simulink model "robotCICESEneurSECcorrGamGA3Wvlt2"  (R2015a)
settings: Solver=ode5  StartTime=0.0  StopTime=200  FixedStep=2.5e-4  MinStep=2.5e-5  RelTol=1e-3
undefined symbols (not defined in the file): F1, F10, F11, F12, F13, F14, F15, F16, F17, F18, F19, F2, F20, F3, F4, F5, F6, F7, F8, F9, Vfinal, Wfinal
libraries: fuzblock x2, simulink_extras x2, simulink x1
settings Model: SimulationMode=accelerator  CovSFcnEnable=off  Creator=Andres Othon  LastModifiedBy=Elothron02
settings DataIOCC: LimitDataPoints=off
settings DebuggingCC: SolverPrmCheckMsg=warning

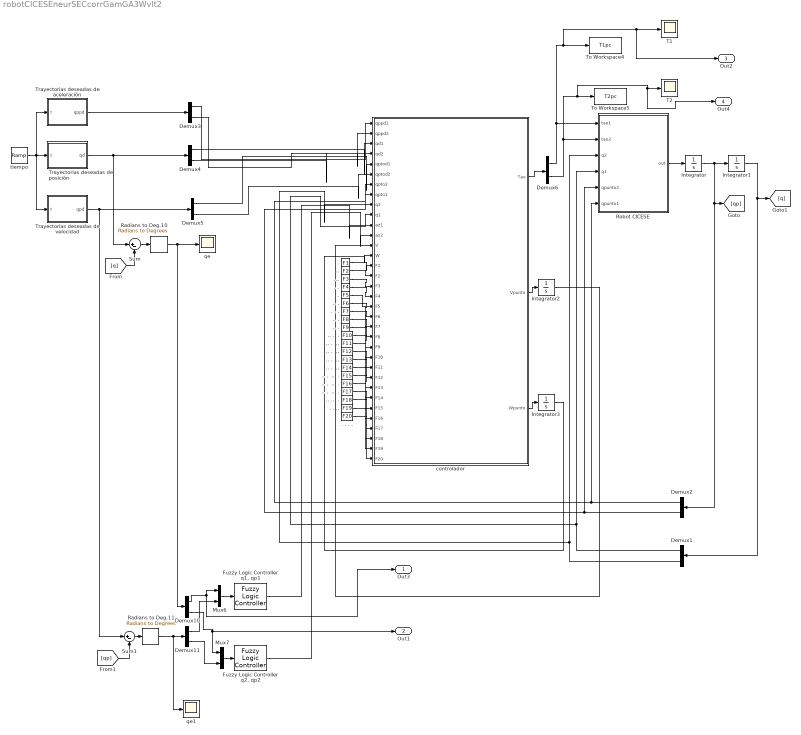
== system robotCICESEneurSECcorrGamGA3Wvlt2 ==
  . : Constant  Value=F1
  ".  " : Constant  Value=F5
  . . : Constant  Value=F4
  . . . : Constant  Value=F7
  ". . . . " : Constant  Value=F20
  ". . .. " : Constant  Value=F19
  .. : Constant  Value=F2
  .. . : Constant  Value=F6
  ".. . " : Constant  Value=F8
  ".. .  " : Constant  Value=F9
  .. .  . : Constant  Value=F10
  .. .  .. : Constant  Value=F11
  ".. .  .. " : Constant  Value=F12
  ".. .  ..  " : Constant  Value=F13
  ".. .  ..   " : Constant  Value=F14
  .. .  ..  . : Constant  Value=F15
  ".. .  ..  . " : Constant  Value=F16
  ".. .  ..  .  " : Constant  Value=F17
  .. ..  . : Constant  Value=F18
  ... : Constant  Value=F3
  Demux{1..6,10..11} (8 alike) : Demux  Outputs=2
  "Fuzzy Logic Controller q1, qp1" : fuzblock/Fuzzy Logic  Controller  fis=['robCICESEq1PREcompGA1xy.fis']
  "Fuzzy Logic Controller q2, qp2" : fuzblock/Fuzzy Logic  Controller  fis=['prub1c.fis']
  Integrator : Integrator
  Integrator1 : Integrator
  Integrator2 : Integrator  InitialCondition=Vfinal%+0.15*randn(7,20)
  Integrator3 : Integrator  InitialCondition=Wfinal%+0.17*randn(20,2)
  Mux6 : Mux  Inputs=2
  Mux7 : Mux  Inputs=2
  Radians to Deg.10 : simulink_extras/Transformations/Radians to Degrees
  Radians to Deg.11 : simulink_extras/Transformations/Radians to Degrees
  Robot CICESE : MATLAB Function  TreatAsAtomicUnit=on
  Sum : Sum  Inputs=|+-
  Sum1 : Sum  Inputs=|+-
  T1 : Scope
      settings: YMin=-125  YMax=175  SaveName=ScopeData2
  T2 : Scope
      settings: TimeRange=10  YMin=-15  YMax=15  SaveName=ScopeData3
  To Workspace4 : ToWorkspace  VariableName=T1pc  SampleTime=-1
  To Workspace5 : ToWorkspace  VariableName=T2pc  SampleTime=-1
  Trayectorias deseadas de aceleración : MATLAB Function  TreatAsAtomicUnit=on
  Trayectorias deseadas de posición : MATLAB Function  TreatAsAtomicUnit=on
  Trayectorias deseadas de velocidad : MATLAB Function  TreatAsAtomicUnit=on
  controlador : MATLAB Function  TreatAsAtomicUnit=on
  qe : Scope
      settings: TimeRange=20  YMax=90  SaveName=ScopeData4
  qe1 : Scope
      settings: TimeRange=20  YMax=90
  tiempo : simulink/Sources/Ramp  slope=1  start=0  X0=0
  Out3 : Outport
  Out1 : Outport  Port=2
  Out2 : Outport  Port=3
  Out4 : Outport  Port=4
  wires:
  Robot CICESE/1(out) -> Integrator/1
  Integrator/1 -> Integrator1/1, [qp], Demux2/1
  Integrator1/1 -> Demux1/1, [q]
  Demux2/1 -> Robot CICESE/6(qpunto1), controlador/8(qpto1)
  Demux2/2 -> Robot CICESE/5(qpunto2), controlador/7(qpto2)
  Demux1/1 -> Robot CICESE/4(q1), controlador/10(q1)
  Demux1/2 -> Robot CICESE/3(q2), controlador/9(q2)
  Demux3/1 -> controlador/1(qppd1)
  Demux3/2 -> controlador/2(qppd2)
  Demux4/1 -> controlador/3(qd1)
  Demux4/2 -> controlador/4(qd2)
  Demux5/1 -> controlador/5(qptod1)
  Demux5/2 -> controlador/6(qptod2)
  controlador/1(Tao) -> Demux6/1
  Demux6/2 -> Robot CICESE/2(tao2), Out4/1, T2/1, To Workspace5/1
  Demux6/1 -> Robot CICESE/1(tao1), Out2/1, T1/1, To Workspace4/1
  [q] -> Sum/2
  [qp] -> Sum1/2
  Demux10/1 -> Out3/1, Mux6/1
  Demux11/1 -> Mux6/2
  Demux10/2 -> Out1/1, Mux7/1
  Demux11/2 -> Mux7/2
  Mux6/1 -> "Fuzzy Logic Controller q1, qp1"/1
  Mux7/1 -> "Fuzzy Logic Controller q2, qp2"/1
  Sum/1 -> Radians to Deg.10/1
  Sum1/1 -> Radians to Deg.11/1
  Radians to Deg.10/1 -> qe/1, Demux10/1
  Radians to Deg.11/1 -> qe1/1, Demux11/1
  "Fuzzy Logic Controller q1, qp1"/1 -> controlador/11(az1)
  "Fuzzy Logic Controller q2, qp2"/1 -> controlador/12(az2)
  controlador/2(Vpunto) -> Integrator2/1
  controlador/3(Wpunto) -> Integrator3/1
  Trayectorias deseadas de aceleración/1(qppd) -> Demux3/1
  Trayectorias deseadas de posición/1(qd) -> Demux4/1, Sum/1
  Trayectorias deseadas de velocidad/1(qpd) -> Demux5/1, Sum1/1
  tiempo/1 -> Trayectorias deseadas de aceleración/1(t), Trayectorias deseadas de posición/1(t), Trayectorias deseadas de velocidad/1(t)
  Integrator3/1 -> controlador/14(W)
  Integrator2/1 -> controlador/13(V)
  ./1 -> controlador/15(F1)
  ../1 -> controlador/16(F2)
  .../1 -> controlador/17(F3)
  . ./1 -> controlador/18(F4)
  ".  "/1 -> controlador/19(F5)
  .. ./1 -> controlador/20(F6)
  . . ./1 -> controlador/21(F7)
  ".. . "/1 -> controlador/22(F8)
  ".. .  "/1 -> controlador/23(F9)
  .. .  ./1 -> controlador/24(F10)
  .. .  ../1 -> controlador/25(F11)
  ".. .  .. "/1 -> controlador/26(F12)
  ".. .  ..  "/1 -> controlador/27(F13)
  ".. .  ..   "/1 -> controlador/28(F14)
  .. .  ..  ./1 -> controlador/29(F15)
  ".. .  ..  . "/1 -> controlador/30(F16)
  ".. .  ..  .  "/1 -> controlador/31(F17)
  .. ..  ./1 -> controlador/32(F18)
  ". . .. "/1 -> controlador/33(F19)
  ". . . . "/1 -> controlador/34(F20)

== matlab function robotCICESEneurSECcorrGamGA3Wvlt2/Trayectorias deseadas de posición ==
  data: t input; qd output
function qd = fcn(t)
%#codegen

qd1 = pi/2 + pi/4*(1 - exp(-2*t^3)) + pi/18*(1 - exp(-2*t^3))*sin(15*t);
qd2 = pi/2 + pi/3*(1 - exp(-1.8*t^3)) + 25*pi/36*(1 - exp(-1.8*t^3))*sin(3.5*t);
qd = [qd1; qd2];

== matlab function robotCICESEneurSECcorrGamGA3Wvlt2/Robot CICESE ==
  data: tao1 input; tao2 input; q2 input; q1 input; qpunto2 input; qpunto1 input; out output
function out = RobotCICESE(tao1, tao2,  q2, q1, qpunto2, qpunto1)
%programa para modelar un robot de 2 grados de libertad, este programa interactua con
%simulink(PDg.mdl). Notar que este programa es una funcion la cual encapsulamos en
%un bloque de simulink(MATLAB function).

% ----ASIGNACION DE VARIABLES----
%variables asignadas a los datos recibidos en el vector de entrada x(n)
%ademas son variables locales, es decir no afectan al archivo de simulink.

%x(2)=posicion angular de la articulaciom 1, radians.
%x(1)=velocidad angular de la articulaciom 1, radianes/segundo.
%x(5)=posicion angular de la articulaciom 2, radians.
%x(6)=velocidad angular de la articulaciom 2, radianes/segundo.
%x(3)=Par motor 1.
%x(4)=Par motor 2.
out = zeros(2,1);
q=[q1; q2];
qpto=[qpunto1; qpunto2];
tao= [tao1; tao2];
%qdpp=[x(7); x(9)];
%qdp=[x(8); x(10)];

% Valores de los parametros del Robot:
gr= 9.81;       % Gravedad (m/seg2)
%m1= 23.902;    % masa eslabon 1 (Kg).
%m2= 3.880;     % masa eslabon 2 (Kg). 
%l1= 0.45;      % longitud eslabon 1 (mts).
%l2= 0.45;      % longitud eslabon 1 (mts).
%lc1=0.091;     % Centro de masa eslabon 1(mts).
%lc2=0.048;     % Centro de masa eslabon 2(mts).
%I1= 1.266;     % Inercia eslabon 1 Kg-m2
%I2= 0.093;     % Inercia eslabon 2 Kg-m2
b1= 2.288;     % Coeficiente de friccion viscosa eslabon 1 (Nm-seg).
b2= 0.175;     % Coeficiente de friccion viscosa eslabon 2 (Nm-seg).

%Calcular las Matrices y Vectores M, C, g y f.
  M=[2.351+0.168.*cos(q(2))  0.102+0.084.*cos(q(2));  0.102+0.084.*cos(q(2))  0.102];
  C=[-0.168*sin(q(2)).*qpto(2)  -0.084.*sin(q(2)).*qpto(2); 0.084.*sin(q(2)).*qpto(1)  0];
  g=[gr.*(3.921.*sin(q(1)) + 0.186.*sin(q(1)+q(2)));  0.186.*gr.*sin(q(1)+q(2))];

%Coeficiente de friccion de Coulomb eslabon 1 (Nm).
  if qpto(1)<0.0
     fc1= -8.049;   
  else
     if qpto(1)>0.0 fc1=7.17; else fc1= 0.0; end
  end

  % Coeficiente de friccion de Coulomb eslabon 2(Nm).
  if qpto(2)<0.0
     fc2= -1.734;   % Coeficiente de friccion de Coulomb eslabon 2(Nm).
  else
     if qpto(2)>0.0 fc2=1.734; else fc2= 0.0; end
  end
  % Friccion de Coulomb
  fc=[fc1; fc2];

  % Friccion Viscosa
  fv=[b1.*qpto(1); b2.*qpto(2)];
tcgf = zeros(2,1);
  
% CALCULO DE LAS DERIVADAS
tcgf=tao - (C*qpto) - g - fv -fc;
qpp=inv(M)*tcgf;


% Salida
out=qpp;

== matlab function robotCICESEneurSECcorrGamGA3Wvlt2/Trayectorias deseadas de velocidad ==
  data: t input; qpd output
function qpd = fcn(t)
%#codegen

qpd1 =  6*pi/4*t^2*exp(-2*t^3) + 6*pi/18*t^2*exp(-2*t^3)*sin(15*t)+ 15*pi/18*(1 - exp(-2*t^3))*cos(15*t);
qpd2 =  5.4*pi/3*t^2*exp(-1.8*t^3) + 5.4*25*pi/36*t^2*exp(-1.8*t^3)*sin(3.5*t)+ 3.5*25*pi/36*(1 - exp(-1.8*t^3))*cos(3.5*t);

qpd = [qpd1; qpd2];

== matlab function robotCICESEneurSECcorrGamGA3Wvlt2/Trayectorias deseadas de aceleración ==
  data: t input; qppd output
function qppd = fcn(t)
%#codegen

qppd1 = 12*(pi/4)*t*exp(-2*t^3) - 36*pi/4*(t^4)*exp(-2*t^3) + 12*pi/18*t*exp(-2*t^3)*sin(15*t) - 36*pi/18*(t^4)*exp(-2*t^3)*sin(15*t) +12*pi/18*(t^2)*exp(-2*t^3)*cos(15*t)*15 - pi/18*(1-exp(-2*t^3))*sin(15*t)*225;

qppd2 = 10.8*pi/3*t*exp(-1.8*t^3)-29.2*pi/3*(t^4)*exp(-1.8*t^3)+10.8*25*pi/36*t*exp(-1.8*t^3)*sin(3.5*t) - 29.2*25*pi/36*(t^4)*exp(-1.8*t^3)*sin(3.5*t) + 10.8*25*pi/36*(t^2)*exp(-1.8*t^3)*cos(3.5*t)*3.5 - 25*pi/36*(1-exp(-1.8*t^3))*sin(3.5*t)*12.25;

qppd = [qppd1; qppd2];

== matlab function robotCICESEneurSECcorrGamGA3Wvlt2/controlador ==
  data: Tao output; qppd1 input; qppd2 input; qd1 input; qd2 input; qptod1 input; qptod2 input; qpto2 input; qpto1 input; q2 input; q1 input; az1 input; az2 input; V input; Vpunto output; W input; Wpunto output; F1 input; F2 input; F3 input; F4 input; F5 input; F6 input; F7 input; F8 input; F9 input; F10 input; F11 input; F12 input; F13 input; F14 input; F15 input; F16 input; F17 input; F18 input; F19 input; F20 input
function [Tao, Vpunto, Wpunto] = controlador(qppd1,qppd2, qd1,qd2,qptod1,qptod2, qpto2, qpto1, q2, q1, az1,az2, V, W, F1, F2, F3, F4, F5, F6, F7, F8, F9, F10, F11, F12, F13, F14, F15, F16, F17, F18, F19, F20)

N = 7;
n = 2;
ele = 20;
Tao = zeros(2,1);
Vpunto = zeros(N,ele);
Wpunto = zeros(ele,n);
%alpha =3.69;%1.7;
alpha = 3.1;
%gamma = 1;
delta=0.5;

%kv = [91*1.1 ;13.9*0.4];
%kp = [33*2.3; 5.5*0.89];

R = diag([ 19.6851,    3.7174,    6.8267,    4.0824,    8.2604,    1.5684,    3.6767]);
%R(2,2) = 0.2;
F = 11*diag([F1, F2, F3, F4, F5, F6, F7, F8, F9, F10, F11, F12, F13, F14, F15, F16, F17, F18, F19, F20]); %F1*eye(20); %0.5*eye(20);
%F(2,2) = 0.1;
qppd = [qppd1;qppd2];
qd = [qd1; qd2];
qptod=[qptod1; qptod2];
qpto=[qpto1; qpto2];
q=[q1; q2];
xd = [1; qd; qptod; qppd];


e = qd - q;
epto = qptod - qpto;

r = epto + alpha*tanh(e);%gamma*e);
sigmaprima1= transpose(V)*xd;
                                                % sigmaprima2 = sech(sigmaprima1).^2;
                                                
sigmaprima = diag(-sigmaprima1.*exp((-sigmaprima1.^2)/2).*(3-sigmaprima1.^2)); %derivada de la wavelet exponencial


sigma = (1-sigmaprima1.^2).*exp((-sigmaprima1.^2)/2);%wavelet sombrero mexicano

Vpunto = R*xd*transpose(r)*transpose(W)*sigmaprima; %corrección del artículo 
                                                                                       % se cambió W por W transpuesta
Wpunto = F*(sigma  -  sigmaprima*sigmaprima1 )*transpose(r);
az = [az1;az2];
%Tao = kp.*tanh(gamma*e) + kv.*epto + delta*sign(r) + transpose(W)*sigma;
Tao = az + delta*sign(r) + transpose(W)*sigma;
